simulink subsystem "Robot_SubSystem"  (R2020b)
settings: Solver=VariableStepAuto  StartTime=0.0  StopTime=10.0  RelTol=1e-3
settings Model: Creator=umberto  LastModifiedBy=Musta

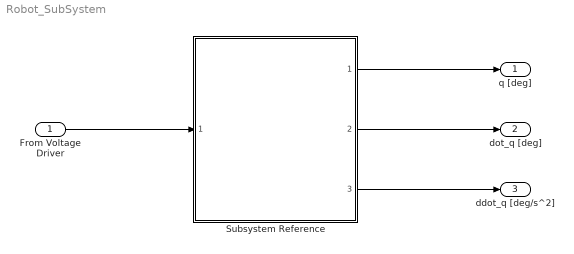
== system Robot_SubSystem ==
  From Voltage Driver : Inport
  Subsystem Reference : Subsystem  ReferencedSubsystem=Electromechanical_SubSystem
  q [deg] : Outport
  dot_q [deg] : Outport  Port=2
  ddot_q [deg/s^2] : Outport  Port=3
  wires:
  From Voltage Driver/1 -> Subsystem Reference/1
  Subsystem Reference/2 -> dot_q [deg]/1
  Subsystem Reference/3 -> ddot_q [deg/s^2]/1
  Subsystem Reference/1 -> q [deg]/1
